simulink model "eval_nets"  (R2021b)
settings: Solver=VariableStepAuto  StartTime=0.0  StopTime=10.0  RelTol=1e-3
settings Model: Creator=Julius  LastModifiedBy=Julius

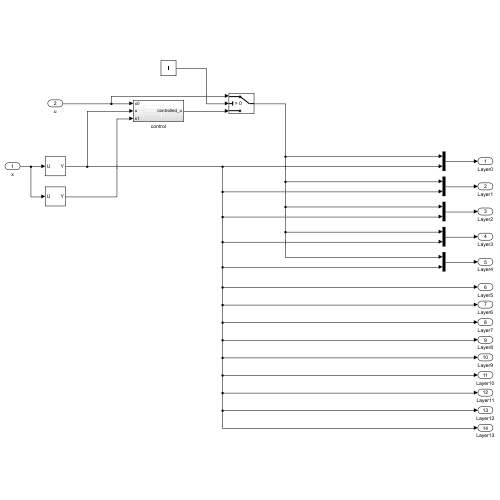
[thumbnail: Simulink's stored preview of the top-level diagram]
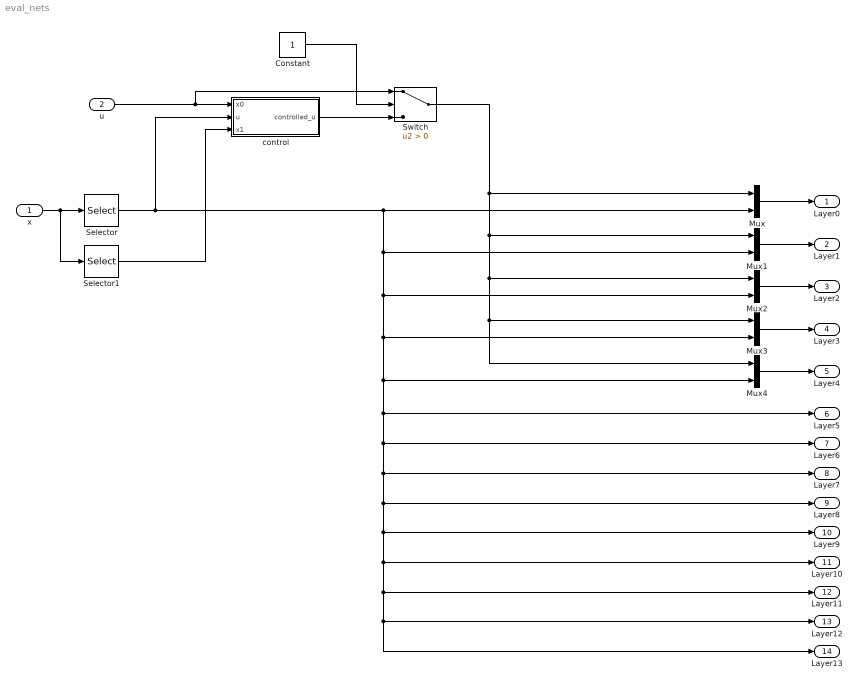
== system eval_nets ==
  x : Inport  PortDimensions=14
  u : Inport  Port=2
  Constant : Constant
  Mux{,1..4} (5 alike) : Mux  Inputs=2
  Selector : Selector  IndexMode=Zero-based  InputPortWidth=14  IndexOptions=Index vector (dialog)  Indices=[1 1]  OutputSizes=1
  Selector1 : Selector  IndexMode=Zero-based  InputPortWidth=14  IndexOptions=Index vector (dialog)  Indices=[2 2]  OutputSizes=1
  Switch : Switch  Criteria=u2 > Threshold
  control : Subsystem
  Layer0 : Outport  OutDataTypeStr=double  PortDimensions=2
  Layer1 : Outport  Port=2  OutDataTypeStr=double  PortDimensions=2
  Layer2 : Outport  Port=3  OutDataTypeStr=double  PortDimensions=2
  Layer3 : Outport  Port=4  OutDataTypeStr=double  PortDimensions=2
  Layer4 : Outport  Port=5  OutDataTypeStr=double  PortDimensions=2
  Layer5 : Outport  Port=6  OutDataTypeStr=double  PortDimensions=1
  Layer6 : Outport  Port=7  OutDataTypeStr=double  PortDimensions=1
  Layer7 : Outport  Port=8  OutDataTypeStr=double  PortDimensions=1
  Layer8 : Outport  Port=9  OutDataTypeStr=double  PortDimensions=1
  Layer9 : Outport  Port=10  OutDataTypeStr=double  PortDimensions=1
  Layer10 : Outport  Port=11  OutDataTypeStr=double  PortDimensions=1
  Layer11 : Outport  Port=12  OutDataTypeStr=double  PortDimensions=1
  Layer12 : Outport  Port=13  OutDataTypeStr=double  PortDimensions=1
  Layer13 : Outport  Port=14  OutDataTypeStr=double  PortDimensions=1
  wires:
  Mux/1 -> Layer0/1
  Mux1/1 -> Layer1/1
  Mux3/1 -> Layer3/1
  Mux2/1 -> Layer2/1
  Mux4/1 -> Layer4/1
  Switch/1 -> Mux4/1, Mux3/1, Mux2/1, Mux1/1, Mux/1
  Selector/1 -> Layer5/1, Layer6/1, Layer7/1, Layer8/1, Layer9/1, Layer10/1, Layer11/1, Layer12/1, Layer13/1, Mux4/2, Mux3/2, Mux2/2, Mux1/2, Mux/2, control/2(u)
  x/1 -> Selector1/1, Selector/1
  u/1 -> Switch/1, control/1(x0)
  Selector1/1 -> control/3(x1)
  control/1(controlled_u) -> Switch/3
  Constant/1 -> Switch/2

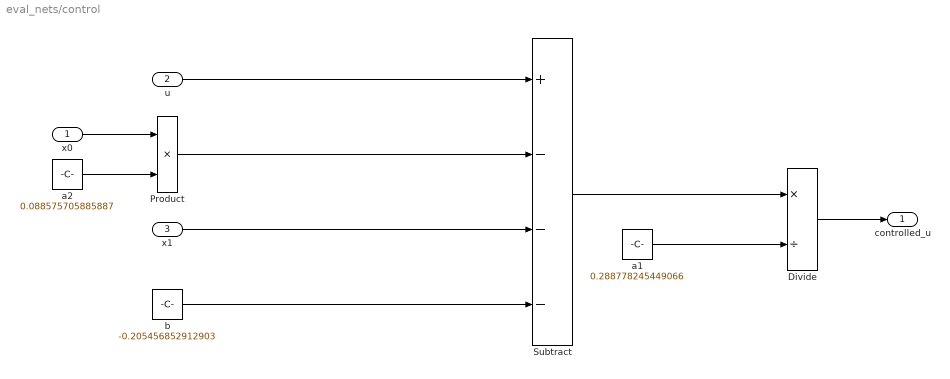
== system eval_nets/control ==
  x0 : Inport
  u : Inport  Port=2
  x1 : Inport  Port=3
  Divide : Product  Inputs=*/
  Product : Product
  Subtract : Sum  Inputs=+---
  a1 : Constant  Value=0.288778245449066
  a2 : Constant  Value=0.088575705885887
  b : Constant  Value=-0.205456852912903
  controlled_u : Outport
  wires:
  x0/1 -> Product/1
  a2/1 -> Product/2
  u/1 -> Subtract/1
  Product/1 -> Subtract/2
  x1/1 -> Subtract/3
  b/1 -> Subtract/4
  Subtract/1 -> Divide/1
  a1/1 -> Divide/2
  Divide/1 -> controlled_u/1
